simulink model "lookupTableDynamic_TestGen29"  (R2017b)
settings: Solver=FixedStepDiscrete  StartTime=0.0  StopTime=10.0  RelTol=1e-3
libraries: simulink x1
settings Model: Creator=ktrinh  LastModifiedBy=ktrinh
settings DebuggingCC: ParameterOverflowMsg=none

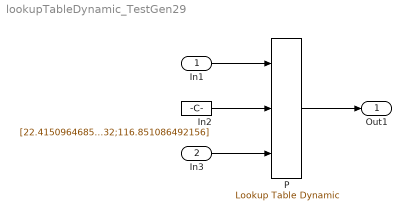
== system lookupTableDynamic_TestGen29 ==
  In1 : Inport  OutMin=20.4151  OutMax=119  OutDataTypeStr=int16  PortDimensions=1
  In3 : Inport  Port=2  PortDimensions=5
  In2 : Constant  Value=[22.4150964685075;41.4607457614945;83.7259479489399;98.8912266634632;116.851086492156]  OutDataTypeStr=int16
  P : simulink/Lookup Tables/Lookup Table Dynamic  LookUpMeth=Use Input Below  OutDataType=fixdt('single')  OutScaling=[]  OutputDataTypeScalingMode=Specify via dialog  OutDataTypeStr=single  RndMeth=Convergent  DoSatur=on
      settings: SourceProductName=Simulink
  Out1 : Outport
  wires:
  In1/1 -> P/1
  In2/1 -> P/2
  In3/1 -> P/3
  P/1 -> Out1/1
